simulink library "F3M_commonLib"  (R2023b)
settings: Solver=VariableStepAuto  StartTime=0.0  StopTime=10.0  RelTol=1e-3
undefined symbols (not defined in the file): entity, F3_getArrayPos, F3_getLossFilter, F3_ptableToArray, F3_ptableToGain, getIsoVec, isoelestring, m, n, Periodicity, pulsewidth, readAttrib, ressize, updateCurrentEProperties, updateInv
libraries: $bdroot x5
(part 2 of 2)

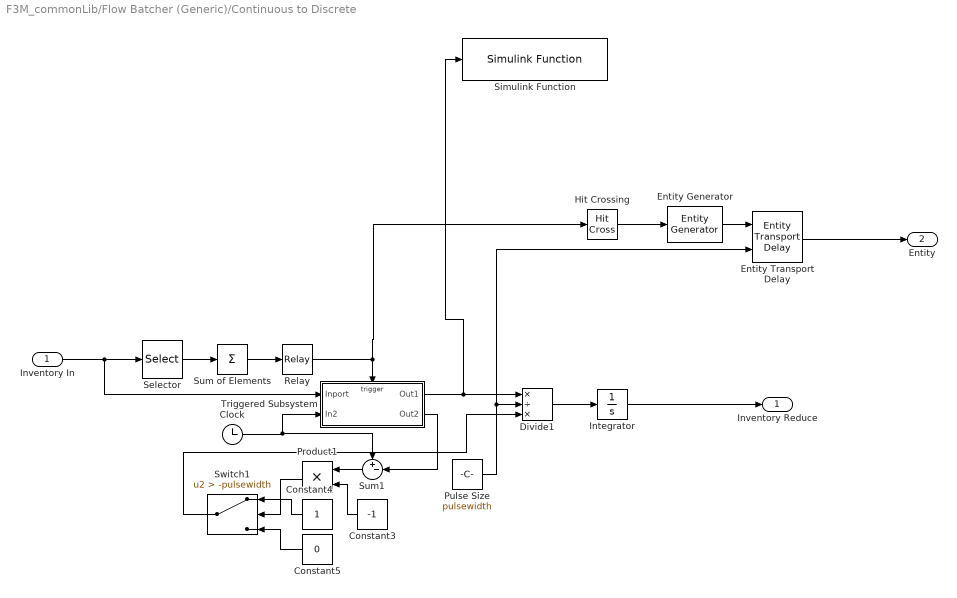
== system F3M_commonLib/Flow Batcher (Generic)/Continuous to Discrete  ==
  Inventory In : Inport
  Clock : Clock
  Constant3 : Constant  Value=-1
  Constant4 : Constant
  Constant5 : Constant  Value=0
  Divide1 : Product  Inputs=*/*
  Entity Transport Delay : EntityTransportDelay  InputPortMessageModes=m,n  OutputPortMessageModes=m
  Entity Generator : EntityGenerator  InputPortMessageModes=m  OutputPortMessageModes=m  GenerationMethod=Event-based  GenerateAction=entity.isovec = updateIsovec();  AttributeName=isovec|auxparam  AttributeInitialValue=zeros(1677,1)|1  EntityType=Structured  EntityTypeName=Entity
      settings: InputPortMap=u0
  Hit Crossing : HitCross  OutputPortMessageModes=m  HitCrossingOffset=1  HitCrossingDirection=rising  HitCrossingOutputType=Message
  Integrator : Integrator
  Product1 : Product
  Pulse Size : Constant  Value=pulsewidth
  Relay : Relay  OnSwitchValue=size+ressize  OffSwitchValue=size+ressize-eps
  Selector : Selector  InputPortWidth=1677  IndexOptions=Index vector (dialog)  Indices=F3_getArrayPos(isoelestring)  OutputSizes=1
  Simulink Function : $bdroot/Continuous to Discrete/Simulink Function  SystemSampleTime=-1  VariantActivationTime=update diagram  AllowFlexibleInterface=on  Latency=0  AutoFrameSizeCalculation=off
  Sum of Elements : Sum  Inputs=+
  Sum1 : Sum  Inputs=+-|
  Switch1 : Switch  Criteria=u2 > Threshold  Threshold=-pulsewidth  SaturateOnIntegerOverflow=off  InputSameDT=off
      settings: AttributesFormatString=-pulseSize
  Triggered Subsystem : Subsystem  AncestorBlock=F3M_commonLib/Continuous to Discrete/Triggered Subsystem  TreatAsAtomicUnit=on
  Inventory Reduce : Outport
  Entity : Outport  Port=2
  wires:
  Clock/1 -> Sum1/1, Triggered Subsystem/2(In2)
  Sum of Elements/1 -> Relay/1
  Constant4/1 -> Switch1/1
  Integrator/1 -> Inventory Reduce/1
  Hit Crossing/1 -> Entity Generator/1
  Pulse Size/1 -> Divide1/2, Entity Transport Delay/2
  Switch1/1 -> Divide1/3
  Constant5/1 -> Switch1/3
  Product1/1 -> Switch1/2
  Constant3/1 -> Product1/2
  Inventory In/1 -> Triggered Subsystem/1(Inport), Selector/1
  Divide1/1 -> Integrator/1
  Triggered Subsystem/2(Out2) -> Sum1/2
  Sum1/1 -> Product1/1
  Selector/1 -> Sum of Elements/1
  Relay/1 -> Hit Crossing/1, Triggered Subsystem/Trigger
  Triggered Subsystem/1(Out1) -> Simulink Function/1, Divide1/1
  Entity Generator/1 -> Entity Transport Delay/1
  Entity Transport Delay/1 -> Entity/1

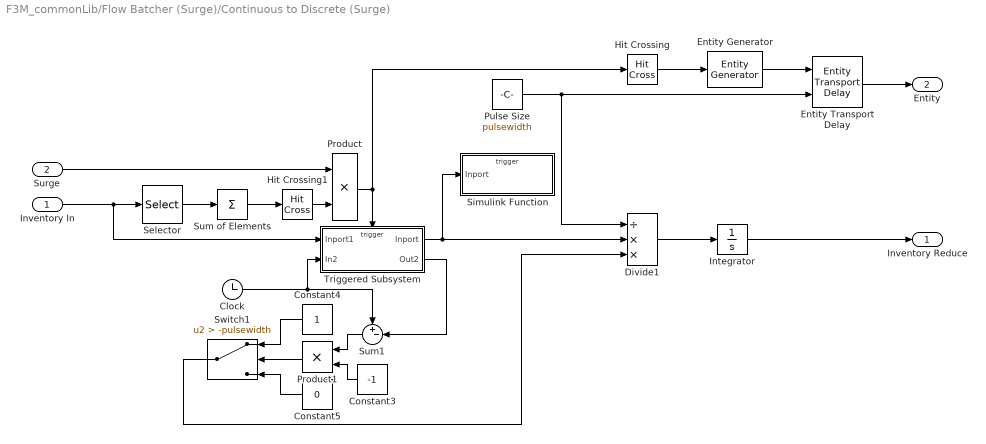
== system F3M_commonLib/Flow Batcher (Surge)/Continuous to Discrete (Surge) ==
  Inventory In : Inport
  Surge : Inport  Port=2
  Clock : Clock
  Constant3 : Constant  Value=-1
  Constant4 : Constant
  Constant5 : Constant  Value=0
  Divide1 : Product  Inputs=/**
  Entity Transport Delay : EntityTransportDelay  InputPortMessageModes=m,n  OutputPortMessageModes=m
  Entity Generator : EntityGenerator  InputPortMessageModes=m  OutputPortMessageModes=m  GenerationMethod=Event-based  GenerateAction=entity.isovec = updateIsovec();  AttributeName=isovec|auxparam  AttributeInitialValue=zeros(1677,1)|1  EntityType=Structured  EntityTypeName=Entity
      settings: InputPortMap=u0
  Hit Crossing : HitCross  OutputPortMessageModes=m  HitCrossingOffset=1  HitCrossingDirection=rising  HitCrossingOutputType=Message
  Hit Crossing1 : HitCross  HitCrossingOffset=size+ressize  HitCrossingDirection=rising
  Integrator : Integrator
  Product : Product
  Product1 : Product
  Pulse Size : Constant  Value=pulsewidth
  Selector : Selector  InputPortWidth=1677  IndexOptions=Index vector (dialog)  Indices=F3_getArrayPos(isoelestring)  OutputSizes=1
  Simulink Function : Subsystem  TreatAsAtomicUnit=on
  Sum of Elements : Sum  Inputs=+
  Sum1 : Sum  Inputs=+-|
  Switch1 : Switch  Criteria=u2 > Threshold  Threshold=-pulsewidth  SaturateOnIntegerOverflow=off  InputSameDT=off
      settings: AttributesFormatString=-pulseSize
  Triggered Subsystem : Subsystem  TreatAsAtomicUnit=on
  Inventory Reduce : Outport
  Entity : Outport  Port=2
  wires:
  Hit Crossing1/1 -> Product/2
  Pulse Size/1 -> Divide1/1, Entity Transport Delay/2
  Inventory In/1 -> Triggered Subsystem/1(Inport1), Selector/1
  Sum of Elements/1 -> Hit Crossing1/1
  Integrator/1 -> Inventory Reduce/1
  Product1/1 -> Switch1/2
  Surge/1 -> Product/1
  Clock/1 -> Sum1/1, Triggered Subsystem/2(In2)
  Triggered Subsystem/2(Out2) -> Sum1/2
  Sum1/1 -> Product1/1
  Product/1 -> Hit Crossing/1, Triggered Subsystem/Trigger
  Entity Generator/1 -> Entity Transport Delay/1
  Divide1/1 -> Integrator/1
  Switch1/1 -> Divide1/3
  Constant3/1 -> Product1/2
  Hit Crossing/1 -> Entity Generator/1
  Entity Transport Delay/1 -> Entity/1
  Selector/1 -> Sum of Elements/1
  Constant4/1 -> Switch1/1
  Constant5/1 -> Switch1/3
  Triggered Subsystem/1(Inport) -> Divide1/2, Simulink Function/1(Inport)

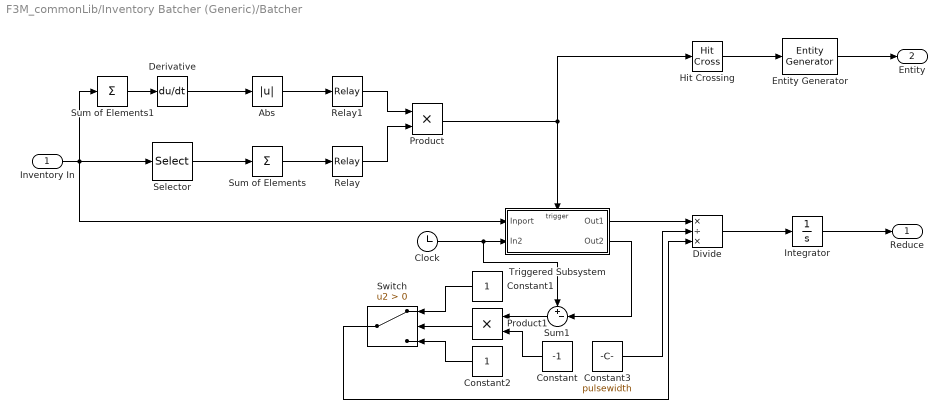
== system F3M_commonLib/Inventory Batcher (Generic)/Batcher ==
  Inventory In : Inport
  Abs : Abs  SaturateOnIntegerOverflow=off
  Clock : Clock
  Constant : Constant  Value=-1
  Constant1 : Constant
  Constant2 : Constant
  Constant3 : Constant  Value=pulsewidth
  Derivative : Derivative
  Divide : Product  Inputs=*/*
  Entity Generator : EntityGenerator  InputPortMessageModes=m  OutputPortMessageModes=m  GenerationMethod=Event-based  GenerateAction=entity.isovec = updateIsovec();  AttributeName=isovec|auxparam  AttributeInitialValue=zeros(1677,1)|1  EntityType=Structured  EntityTypeName=Entity
      settings: InputPortMap=u0
  Hit Crossing : HitCross  HitCrossingOffset=1  HitCrossingDirection=rising  HitCrossingOutputType=Message
  Integrator : Integrator
  Product : Product
  Product1 : Product
  Relay : Relay  OnSwitchValue=size+ressize  OffSwitchValue=size+ressize-eps
  Relay1 : Relay  OffSwitchValue=0  OnOutputValue=0  OffOutputValue=1
  Selector : Selector  InputPortWidth=1677  IndexOptions=Index vector (dialog)  Indices=F3_getArrayPos(isoelestring)  OutputSizes=1
  Sum of Elements : Sum  Inputs=+
  Sum of Elements1 : Sum  Inputs=+
  Sum1 : Sum  Inputs=+-|
  Switch : Switch  Criteria=u2 > Threshold  SaturateOnIntegerOverflow=off  InputSameDT=off
  Triggered Subsystem : Subsystem  TreatAsAtomicUnit=on
  Reduce : Outport
  Entity : Outport  Port=2
  wires:
  Inventory In/1 -> Triggered Subsystem/1(Inport), Sum of Elements1/1, Selector/1
  Selector/1 -> Sum of Elements/1
  Sum of Elements/1 -> Relay/1
  Sum of Elements1/1 -> Derivative/1
  Derivative/1 -> Abs/1
  Abs/1 -> Relay1/1
  Relay1/1 -> Product/1
  Relay/1 -> Product/2
  Product/1 -> Triggered Subsystem/Trigger, Hit Crossing/1
  Clock/1 -> Sum1/1, Triggered Subsystem/2(In2)
  Triggered Subsystem/2(Out2) -> Sum1/2
  Sum1/1 -> Product1/1
  Constant/1 -> Product1/2
  Product1/1 -> Switch/2
  Constant2/1 -> Switch/3
  Constant1/1 -> Switch/1
  Triggered Subsystem/1(Out1) -> Divide/1
  Constant3/1 -> Divide/2
  Switch/1 -> Divide/3
  Divide/1 -> Integrator/1
  Integrator/1 -> Reduce/1
  Entity Generator/1 -> Entity/1
  Hit Crossing/1 -> Entity Generator/1

== system F3M_commonLib/Flow Batcher (Generic)/Continuous to Discrete /Triggered Subsystem ==
  Inport : Inport
  In2 : Inport  Port=2
  Trigger : TriggerPort  VariantControl=(inherit)
  Constant : Constant  Value=size
  Divide : Product  Inputs=*/*
  Selector : Selector  InputPortWidth=1677  IndexOptions=Index vector (dialog)  Indices=F3_getArrayPos(isoelestring)  OutputSizes=1
  Sum of Elements : Sum  Inputs=+
  Out1 : Outport
  Out2 : Outport  Port=2
  wires:
  In2/1 -> Out2/1
  Constant/1 -> Divide/3
  Sum of Elements/1 -> Divide/2
  Inport/1 -> Divide/1, Selector/1
  Divide/1 -> Out1/1
  Selector/1 -> Sum of Elements/1

== system F3M_commonLib/Flow Batcher (Surge)/Continuous to Discrete (Surge)/Simulink Function ==
  Inport : Inport
  updateIsovec() : TriggerPort  TriggerType=function-call  IsSimulinkFunction=on  FunctionName=updateIsovec  FunctionVisibility=scoped  VariantControl=(inherit)
  y : ArgOut  DisableCoverage=on  PortDimensions=1677  ArgumentName=y
  wires:
  Inport/1 -> y/1

== system F3M_commonLib/Flow Batcher (Surge)/Continuous to Discrete (Surge)/Triggered Subsystem ==
  Inport1 : Inport
  In2 : Inport  Port=2
  Trigger : TriggerPort  VariantControl=(inherit)
  Constant : Constant  Value=size
  Divide : Product  Inputs=*/*
  Selector : Selector  InputPortWidth=1677  IndexOptions=Index vector (dialog)  Indices=F3_getArrayPos(isoelestring)  OutputSizes=1
  Sum of Elements : Sum  Inputs=+
  Inport : Outport
  Out2 : Outport  Port=2
  wires:
  In2/1 -> Out2/1
  Sum of Elements/1 -> Divide/2
  Divide/1 -> Inport/1
  Inport1/1 -> Divide/1, Selector/1
  Selector/1 -> Sum of Elements/1
  Constant/1 -> Divide/3

== system F3M_commonLib/Inventory Batcher (Generic)/Batcher/Triggered Subsystem ==
  Inport : Inport
  In2 : Inport  Port=2
  Trigger : TriggerPort  VariantControl=(inherit)
  Constant : Constant  Value=size
  Divide : Product  Inputs=*/*
  Selector : Selector  InputPortWidth=1677  IndexOptions=Index vector (dialog)  Indices=F3_getArrayPos(isoelestring)  OutputSizes=1
  Sum of Elements : Sum  Inputs=+
  Out1 : Outport
  Out2 : Outport  Port=2
  wires:
  Inport/1 -> Divide/1, Selector/1
  Selector/1 -> Sum of Elements/1
  Sum of Elements/1 -> Divide/2
  Constant/1 -> Divide/3
  In2/1 -> Out2/1
  Divide/1 -> Out1/1

== matlab function F3M_commonLib/Discrete Material Loss/Simulink Function/MATLAB Function ==
  data: isovec input; y output; lossvec input; replacevec input
function y = fcn(isovec, lossvec, replacevec)

y = isovec;
y = y - y.*lossvec;

diff = isovec - y;
y = y + sum(diff)*replacevec;

== matlab function F3M_commonLib/Discrete to Continuous/Simulink Function/MATLAB Function ==
  data: isovec input; y output
function y = fcn(isovec)

y = isovec;

== matlab function F3M_commonLib/Discrete Material Loss/Simulink Function2/MATLAB Function ==
  data: isovec input; y output; lossfrac input
function y = fcn(isovec, lossfrac)

y = isovec.*lossfrac;

== matlab function F3M_commonLib/Custom Source Generator/Simulink Function/MATLAB Function ==
  data: itemsize input; ptable input; y output
function y = fcn(itemsize,ptable)

y = zeros(1677,1);
y(int16(ptable(1,:))) = ptable(2,:)*itemsize;

== matlab function F3M_commonLib/Entity Process and Hold/Simulink Function/MATLAB Function ==
  data: isovec input; mod_entity output; ptable_array input; etype input
function mod_entity = fcn(isovec,ptable_array,etype)

mod_entity = F3_calculateLossEntities(isovec,ptable_array,etype);

== matlab function F3M_commonLib/Discrete Material Loss/Simulink Function3/MATLAB Function ==
  data: isovec input; lossvec input; y output; replacevec input
function y = fcn(isovec, lossvec, replacevec)


lossT = isovec.*lossvec;

y = sum(lossT)*replacevec;

== matlab function F3M_commonLib/Entity Process and Hold/Subsystem/MATLAB Function ==
  data: isovec input; utype input; y output
function y = fcn(isovec, utype)

persistent inventory

if isempty(inventory)
    inventory = isovec;
else
    if utype == 1 %addition
    inventory = inventory+isovec;
    else %subtraction
    inventory = inventory-isovec;
    end
end




y = inventory;

== matlab function F3M_commonLib/Entity Hold (Periodic)/Simulink Function/MATLAB Function ==
  data: isovec input; utype input; y output
function y = fcn(isovec, utype)

persistent inventory

if isempty(inventory)
    inventory = isovec;
else
    if utype == 1 %addition
    inventory = inventory+isovec;
    else %subtraction
    inventory = inventory-isovec;
    end
end




y = inventory;
